simulink model "Line_keeping"  (R2023a)
settings: Solver=ode23tb  StartTime=0.0  StopTime=50  RelTol=1e-3
model workspace (MAT data in the model file):
  BusActorsActors = canlib.Parameter
  BusActorsActors.DataType = 'auto'
  BusActorsActors.Complexity = 'real'
  BusActorsActors.Dimensions = [0 0]
values from neighbouring files (symbols this model uses):
  Cf = 19000    [L_1_init.m]    (also in calc_KMax.m; calc_Kmin.m; init.m; init_h2.m)
  Cr = 33000    [L_1_init.m]    (also in calc_KMax.m; calc_Kmin.m; init.m; init_h2.m)
  Iz = 2875    [L_1_init.m]    (also in calc_KMax.m; calc_Kmin.m; init.m; init_h2.m)
  Lf = 1.2    [L_1_init.m]    (also in calc_KMax.m; calc_Kmin.m; init.m; init_h2.m)
  Lr = 1.6    [L_1_init.m]    (also in calc_KMax.m; calc_Kmin.m; init.m; init_h2.m)
  m = dim(2)    [H_2_gain.m]    (also in L_1_init.m = 1575; calc_KMax.m = 1575; calc_Kmin.m = 1575; init.m = 1575)
  x_0 = [0 0 0 0]'    [L_1_init.m]    (also in init.m; init_h2.m; init_h8.m)
undefined symbols (not defined in the file or in its folder): driving, sigbuilder_block
libraries: drivingscenarioandsensors x2
settings Model: PacingRate=2  Creator=Utente  LastModifiedBy=csanc
settings SolverCC: AlgebraicLoopSolver=TrustRegion
settings DebuggingCC: UnconnectedInputMsg=warning  UnconnectedOutputMsg=warning  UnconnectedLineMsg=warning
settings ModelReferenceCC: EnableRefExpFcnMdlSchedulingChecks=on
settings RTWCC: DLArmComputeVersion=19.05

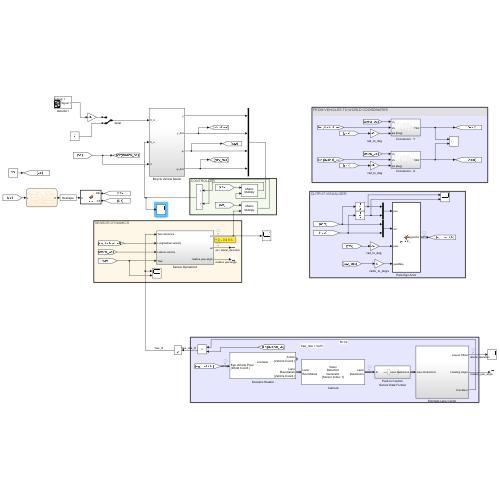
[thumbnail: Simulink's stored preview of the top-level diagram]
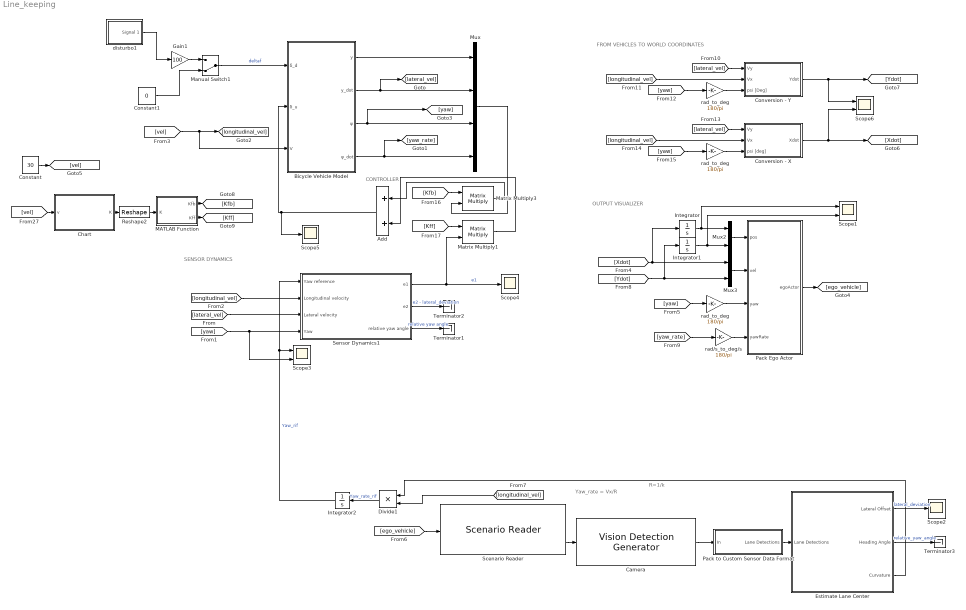
== system Line_keeping ==
  note: R=1/k
  note: Yaw_rate = Vx/R
  note: FROM VEHICLES TO WORLD COORDINATES
  note: SENSOR DYNAMICS
  note: CONTROLLER
  note: OUTPUT VISUALIZER
  Add : Sum
  Bicycle Vehicle Model : Subsystem
  Camera : drivingscenarioandsensors/Vision Detection Generator  SensorIndex=1  DetectorOutput=Lanes only  UpdateInterval=0.1  LaneUpdateInterval=0.01  SensorLocation=[1.9 0]  Height=1.1  Yaw=0  Pitch=0  Roll=0  BusNameSource=Auto  BusName=BusObjectDetections  BusName2Source=Property  BusName2=BusVision  MaxNumDetectionsSource=Property  MaxNumDetections=50  MaxNumLanesSource=Property  MaxNumLanes=2  DetectionCoordinates=Ego Cartesian  SimulateUsing=Interpreted execution  MaxRange=50  BoundingBoxAccuracy=10  ProcessNoiseIntensity=5  MaxSpeed=50  MaxAllowedOcclusion=0.5  MinObjectImageSize=[15 15]  DetectionProbability=0.9  FalsePositivesPerImage=0.1  MinLaneImageSize=[20 3]  LaneBoundaryAccuracy=3  HasNoise=on  InitialSeedSource=Repeatable  InitialSeed=0  UsedSeed=0  ActorProfilesSource=Parameters  ActorProfilesParameters=driving.internal.ActorProfilesParameters  ActorProfilesExpression=[struct('ActorID',1,'ClassID',1,'Length',4.7,'Width',1.8,'Height',1.4,'OriginOffset',[-1.35 0 0],'MeshVertices',[3.7 -0.9 1.4;3.7 0.9 1.4;-1 0.9 1.4;-1 -0.9 1.4;3.7 -0.9 0;3.7 0.9 0;-1 0.9 0;-1 -0.9 0],'MeshFaces',[6 2 1;1 5 6;8 4 3;3 7 8;6 7 3;3 2 6;5 1 4;4 8 5;4 1 2;2 3 4;7 6 5;5 8 7],'RCSPattern',[10 10;10 10],'RCSAzimuthAngles',[-180 180],'RCSElevationAngles',[-90 90])]  Intrinsics=driving.internal.cameraIntrinsics('FocalLength',[800 800],'PrincipalPoint',[320 240],'ImageSize',[480 640],'RadialDistortion',[0 0],'TangentialDistortion',[0 0],'Skew',0)
  Chart : Stateflow chart  TreatAsAtomicUnit=on
  Constant : Constant  Value=30
  Constant1 : Constant  Value=0
  Conversion - X : Subsystem
  Conversion - Y : Subsystem
  Divide1 : Product  Inputs=**
  Estimate Lane Center : Subsystem  VariantControl=v2
  Gain1 : Gain  Gain=100
  Integrator : Integrator
  Integrator1 : Integrator  InitialCondition=-0.02
  Integrator2 : Integrator
  MATLAB Function : MATLAB Function  TreatAsAtomicUnit=on
  Manual Switch1 : ManualSwitch  CurrentSetting=0
  Matrix Multiply1 : Product  Multiplication=Matrix(*)
  Matrix Multiply3 : Product  Multiplication=Matrix(*)
  Mux : Mux
  Mux2 : Mux  Inputs=2
  Mux3 : Mux  Inputs=2
  Pack Ego Actor : MATLAB Function  TreatAsAtomicUnit=on
  Pack to Custom Sensor Data Format : Subsystem
  Reshape2 : Reshape  OutputDimensionality=Customize  OutputDimensions=[1,5]
  Scenario Reader : drivingscenarioandsensors/Scenario Reader  ScenarioSource=From file  ScenarioFileName=D:\Proyecto_vehicle_control\modulo 2\scenario.mat  ScenarioVariableName=scenario  OutputCoordinateSystem=Vehicle coordinates  EgoVehicleSource=Input port  EgoVehicleActorID=1  OrientVehiclesOnRoad=off  OutputEgoVehiclePose=off  OutputEgoVehicleState=off  SampleTime=.1  LaneBoundaryOutput=Ego vehicle lane boundaries  LaneBoundaryDistance=linspace(-150, 150, 101)  LaneBoundaryLocation=Center of lane markings  BusNameSource=Auto  BusName=BusActors  BusNumActorsSource=Scenario  BusNumActors=100  BusName2Source=Auto  BusName2=BusLaneBoundaries  BusNumLaneBoundariesSource=Scenario  BusNumLaneBoundaries=10  BusName3Source=Auto  BusName3=BusEgoActor  BusName4Source=Auto  BusName4=BusEgoState  ShowCoordinateLabels=on  SimulateUsing=Interpreted execution
  Scope1 : Scope  NumInputPorts=2
  Scope2 : Scope
  Scope3 : Scope  NumInputPorts=2
  Scope4 : Scope
  Scope5 : Scope
  Scope6 : Scope  NumInputPorts=2
  Sensor Dynamics1 : Subsystem
  Terminator1 : Terminator
  Terminator2 : Terminator
  Terminator3 : Terminator
  disturbo1 : Subsystem  Tag=STV Subsys  LoadFcn=sigbuilder_block('load');  StartFcn=sigbuilder_block('start');  StopFcn=sigbuilder_block('stop');  ClipboardFcn=sigbuilder_block('clipboard');  mask(Sigbuilder block){tuvar=[0:10]}
      mask help: Simulink:masks:SigbuilderBlock_MD
      mask init:
      | if ~strcmp(get_param(bdroot(gcbh),'SimulationStatus'),'stopped') tuvar = sigbuilder_block('maskInit'); end
      settings: CopyFcn=sigbuilder_block('copy');  DeleteFcn=sigbuilder_block('delete');  ModelCloseFcn=sigbuilder_block('modelClose');  PreSaveFcn=sigbuilder_block('preSave');  PauseFcn=sigbuilder_block('pause');  ContinueFcn=sigbuilder_block('continue');  NameChangeFcn=sigbuilder_block('namechange');  OpenFcn=sigbuilder_block('open',[406.2 255 401.4 229.8 ]);  CloseFcn=sigbuilder_block('close');
      mask Display: plot(0, 0, 100, 100,[2, 2, 32, 32, 2], [68, 8, 8, 68, 68],[32, 2], [38, 38], [32, 19, 2],[53, 60, 44], [32, 17, 17, 2],[16, 16, 31, 31]);txt = getActiveGroup(gcbh);text(2, 100, txt,'verticalAlignment', 'top');
  rad/s_to_deg/s : Gain  Gain=180/pi
  rad_to_deg : Gain  Gain=180/pi
  "rad_to_deg " : Gain  Gain=180/pi
  "rad_to_deg  " : Gain  Gain=180/pi
  wires:
  Bicycle Vehicle Model/1(y) -> Mux/1
  Bicycle Vehicle Model/2(y_dot) -> [lateral_vel], Mux/2
  Bicycle Vehicle Model/4(ψ_dot) -> [yaw_rate], Mux/4
  Mux/1 -> Matrix Multiply3/2
  [longitudinal_vel] -> Sensor Dynamics1/2(Longitudinal velocity)
  [lateral_vel] -> Sensor Dynamics1/3(Lateral velocity)
  [yaw] -> Scope3/2, Sensor Dynamics1/4("Yaw ")
  Mux2/1 -> Pack Ego Actor/1(pos)
  [Xdot] -> Integrator/1, Mux3/1
  Mux3/1 -> Pack Ego Actor/2(vel)
  [yaw] -> "rad_to_deg  "/1
  Pack Ego Actor/1(egoActor) -> [ego_vehicle]
  [yaw_rate] -> rad/s_to_deg/s/1
  "rad_to_deg  "/1 -> Pack Ego Actor/3(yaw)
  [Ydot] -> Integrator1/1, Mux3/2
  rad/s_to_deg/s/1 -> Pack Ego Actor/4(yawRate)
  [lateral_vel] -> Conversion - Y/1(Vy)
  [longitudinal_vel] -> Conversion - Y/2(Vx)
  Conversion - X/1(Xdot) -> [Xdot], Scope6/2
  [yaw] -> rad_to_deg/1
  [yaw] -> "rad_to_deg "/1
  [longitudinal_vel] -> Conversion - X/2(Vx)
  [lateral_vel] -> Conversion - X/1(Vy)
  rad_to_deg/1 -> Conversion - X/3(psi [deg])
  "rad_to_deg "/1 -> Conversion - Y/3(psi [Deg])
  Sensor Dynamics1/3(relative yaw angle) -> Terminator1/1  "relative yaw angle"
  Integrator/1 -> Scope1/1, Mux2/1
  Integrator1/1 -> Scope1/2, Mux2/2
  Camera/1 -> Pack to Custom Sensor Data Format/1(In)
  Scenario Reader/2 -> Camera/1
  Pack to Custom Sensor Data Format/1(Lane Detections) -> Estimate Lane Center/1(Lane Detections)
  [ego_vehicle] -> Scenario Reader/1
  Divide1/1 -> Integrator2/1  "Yaw_rate_rif"
  Add/1 -> Scope5/1, Bicycle Vehicle Model/2(δ_u)
  Bicycle Vehicle Model/3(ψ) -> [yaw], Mux/3
  Estimate Lane Center/3(" Curvature") -> Divide1/1
  Conversion - Y/1(Ydot) -> [Ydot], Scope6/1
  Integrator2/1 -> Scope3/1, Sensor Dynamics1/1(Yaw reference)  "Yaw_rif"
  [longitudinal_vel] -> Divide1/2
  Sensor Dynamics1/2(e2) -> Terminator2/1  "e2 - lateral_deviation"
  Estimate Lane Center/1(Lateral Offset) -> Scope2/1  "lateral_deviation"
  [vel] -> Chart/1(v)
  [vel] -> [longitudinal_vel], Bicycle Vehicle Model/3(V)
  MATLAB Function/1(Kfb) -> [Kfb]
  MATLAB Function/2(Kff) -> [Kff]
  [Kfb] -> Matrix Multiply3/1
  Matrix Multiply3/1 -> Add/1
  [Kff] -> Matrix Multiply1/1
  Sensor Dynamics1/1(e1) -> Scope4/1, Matrix Multiply1/2  "e1"
  Matrix Multiply1/1 -> Add/2
  Chart/1(K) -> Reshape2/1
  Reshape2/1 -> MATLAB Function/1(K)
  Constant/1 -> [vel]
  Constant1/1 -> Manual Switch1/2
  Manual Switch1/1 -> Bicycle Vehicle Model/1(δ_d)  "deltaf"
  disturbo1/1(Signal 1) -> Gain1/1
  Gain1/1 -> Manual Switch1/1
  Estimate Lane Center/2(Heading Angle) -> Terminator3/1  "relative_yaw_angle"

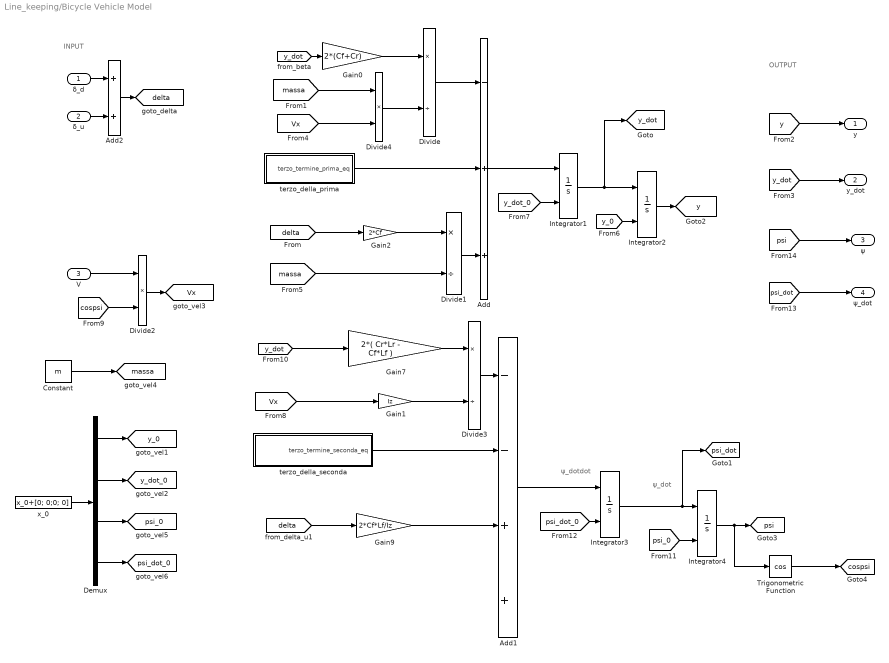
== system Line_keeping/Bicycle Vehicle Model ==
  note: ψ_dot
  note: OUTPUT
  note: INPUT
  note: ψ_dotdot
  δ_d : Inport
  δ_u : Inport  Port=2
  V : Inport  Port=3
  Add : Sum  Inputs=-++
  Add1 : Sum  Inputs=--++
  Add2 : Sum
  Constant : Constant  Value=m
  Demux : Demux
  Divide : Product  Inputs=*/
  Divide1 : Product  Inputs=*/
  Divide2 : Product  Inputs=**
  Divide3 : Product  Inputs=*/
  Divide4 : Product  Inputs=**
  Gain0 : Gain  Gain=2*(Cf+Cr)
  Gain1 : Gain  Gain=Iz
  Gain2 : Gain  Gain=2*Cf
  Gain7 : Gain  Gain="2*( Cr*Lr  - Cf*Lf )"
  Gain9 : Gain  Gain=2*Cf*Lf/Iz
  Integrator1 : Integrator  InitialConditionSource=external
  Integrator2 : Integrator  InitialConditionSource=external
  Integrator3 : Integrator  InitialConditionSource=external
  Integrator4 : Integrator  InitialConditionSource=external  LowerSaturationLimit=0
  Trigonometric Function : Trigonometry  Operator=cos
  terzo_della_prima : Subsystem
  terzo_della_seconda : Subsystem
  "x_0 " : Constant  Value=x_0+[0; 0;0; 0]
  y : Outport
  y_dot : Outport  Port=2
  ψ : Outport  Port=3
  ψ_dot : Outport  Port=4
  tag scope: Vx=global, cospsi=global, delta=global, massa=global, psi=global, psi_0=global, psi_dot=global, psi_dot_0=global, y=global, y_0=global, y_dot=global, y_dot_0=global
  wires:
  [psi] -> ψ/1
  [psi_dot] -> ψ_dot/1
  [psi_dot_0] -> Integrator3/2
  [psi_0] -> Integrator4/2
  [cospsi] -> Divide2/2
  Trigonometric Function/1 -> [cospsi]
  Divide2/1 -> [Vx]
  Integrator4/1 -> [psi], Trigonometric Function/1
  [Vx] -> Gain1/1
  Gain1/1 -> Divide3/2
  Divide3/1 -> Add1/1
  [y_0] -> Integrator2/2
  [y_dot_0] -> Integrator1/2
  Demux/4 -> [psi_dot_0]
  Demux/3 -> [psi_0]
  Integrator2/1 -> [y]
  Integrator1/1 -> [y_dot], Integrator2/1
  Divide1/1 -> Add/3
  [massa] -> Divide1/2
  Divide/1 -> Add/1
  [Vx] -> Divide4/2
  [massa] -> Divide4/1
  Divide4/1 -> Divide/2
  "x_0 "/1 -> Demux/1
  [delta] -> Gain2/1
  Add2/1 -> [delta]
  Gain9/1 -> Add1/3
  terzo_della_seconda/1("terzo_termine_seconda_eq ") -> Add1/2
  Gain2/1 -> Divide1/1
  terzo_della_prima/1("terzo_termine_prima_eq ") -> Add/2
  Demux/2 -> [y_dot_0]
  Demux/1 -> [y_0]
  Constant/1 -> [massa]
  Integrator3/1 -> Integrator4/1, [psi_dot]
  Add/1 -> Integrator1/1
  [y_dot] -> Gain7/1
  [y_dot] -> Gain0/1
  [y_dot] -> y_dot/1
  [y] -> y/1
  [delta] -> Gain9/1
  Gain7/1 -> Divide3/1
  Add1/1 -> Integrator3/1
  Gain0/1 -> Divide/1
  V/1 -> Divide2/1
  δ_u/1 -> Add2/2
  δ_d/1 -> Add2/1

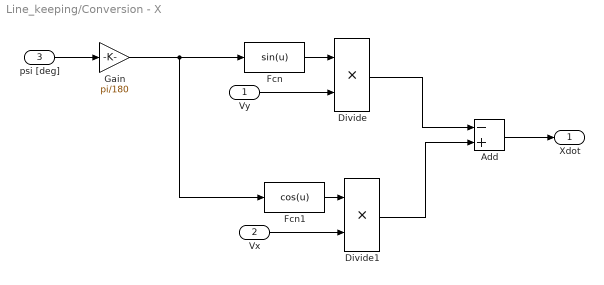
== system Line_keeping/Conversion - X ==
  Vy : Inport
  Vx : Inport  Port=2
  psi [deg] : Inport  Port=3
  Add : Sum  Inputs=-+
  Divide : Product  Inputs=**
  Divide1 : Product  Inputs=**
  Fcn : Fcn  Expr=sin(u)
  Fcn1 : Fcn  Expr=cos(u)
  Gain : Gain  Gain=pi/180
  Xdot : Outport
  wires:
  Gain/1 -> Fcn/1, Fcn1/1
  Add/1 -> Xdot/1
  Divide1/1 -> Add/2
  Vx/1 -> Divide1/2
  Fcn1/1 -> Divide1/1
  Divide/1 -> Add/1
  Vy/1 -> Divide/2
  Fcn/1 -> Divide/1
  psi [deg]/1 -> Gain/1

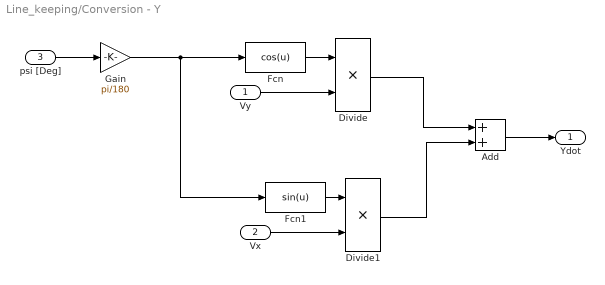
== system Line_keeping/Conversion - Y ==
  Vy : Inport
  Vx : Inport  Port=2
  psi [Deg] : Inport  Port=3
  Add : Sum
  Divide : Product  Inputs=**
  Divide1 : Product  Inputs=**
  Fcn : Fcn  Expr=cos(u)
  Fcn1 : Fcn  Expr=sin(u)
  Gain : Gain  Gain=pi/180
  Ydot : Outport
  wires:
  psi [Deg]/1 -> Gain/1
  Fcn/1 -> Divide/1
  Vy/1 -> Divide/2
  Divide/1 -> Add/1
  Fcn1/1 -> Divide1/1
  Vx/1 -> Divide1/2
  Divide1/1 -> Add/2
  Add/1 -> Ydot/1
  Gain/1 -> Fcn1/1, Fcn/1

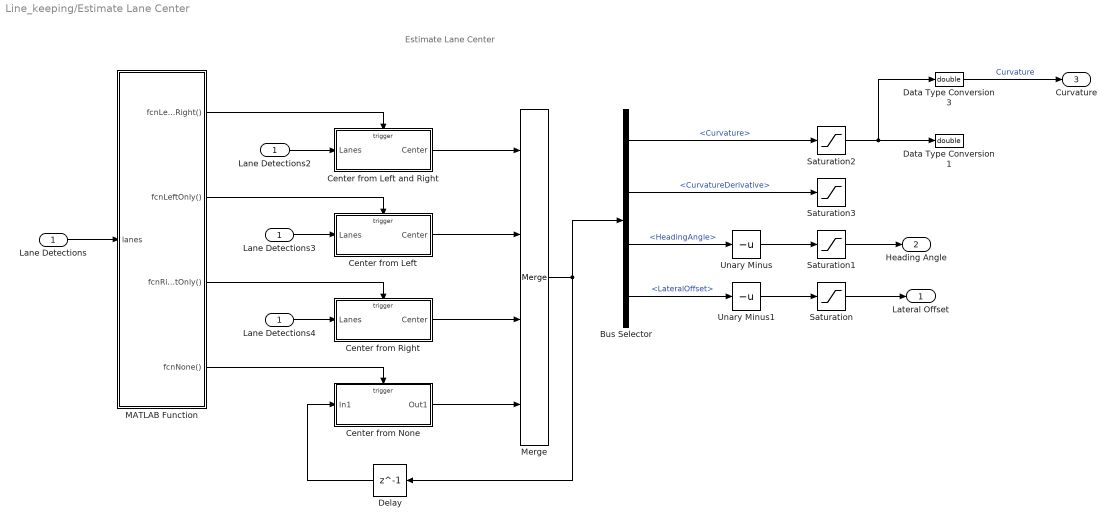
== system Line_keeping/Estimate Lane Center ==
  note: Estimate Lane Center
  Lane Detections : Inport
  Bus Selector : BusSelector  OutputSignals=Curvature,CurvatureDerivative,HeadingAngle,LateralOffset
  Center from Left : Subsystem  TreatAsAtomicUnit=on
  Center from Left and Right : Subsystem  TreatAsAtomicUnit=on
  Center from None : Subsystem  TreatAsAtomicUnit=on
  Center from Right : Subsystem  TreatAsAtomicUnit=on
  Data Type Conversion1 : DataTypeConversion  OutDataTypeStr=double  SaturateOnIntegerOverflow=off  RndMeth=Floor
  Data Type Conversion3 : DataTypeConversion  OutDataTypeStr=double  SaturateOnIntegerOverflow=off  RndMeth=Floor
  Delay : Delay  DelayLength=1
  Lane Detections2 : InportShadow
  Lane Detections3 : InportShadow
  Lane Detections4 : InportShadow
  MATLAB Function : MATLAB Function  TreatAsAtomicUnit=on
  Merge : Merge  Inputs=4
  Saturation : Saturate  UpperLimit=inf
  Saturation1 : Saturate  UpperLimit=0.6  LowerLimit=-0.6
  Saturation2 : Saturate  UpperLimit=0.15  LowerLimit=-0.15
  Saturation3 : Saturate  UpperLimit=0.15  LowerLimit=-0.15
  Unary Minus : UnaryMinus
  Unary Minus1 : UnaryMinus
  Lateral Offset : Outport  VectorParamsAs1DForOutWhenUnconnected=off
  Heading Angle : Outport  Port=2  VectorParamsAs1DForOutWhenUnconnected=off
  " Curvature" : Outport  Port=3  VectorParamsAs1DForOutWhenUnconnected=off
  wires:
  Center from Right/1(Center) -> Merge/3
  Lane Detections3/1 -> Center from Left/1(Lanes)
  Lane Detections4/1 -> Center from Right/1(Lanes)
  MATLAB Function/2(fcnLeftOnly()) -> Center from Left/Trigger
  Center from None/1(Out1) -> Merge/4
  MATLAB Function/1(fcnLeftAndRight()) -> Center from Left and Right/Trigger
  Delay/1 -> Center from None/1(In1)
  Center from Left and Right/1(Center) -> Merge/1
  Lane Detections/1 -> MATLAB Function/1(lanes)
  Lane Detections2/1 -> Center from Left and Right/1(Lanes)
  MATLAB Function/3(fcnRightOnly()) -> Center from Right/Trigger
  MATLAB Function/4(fcnNone()) -> Center from None/Trigger
  Center from Left/1(Center) -> Merge/2
  Merge/1 -> Bus Selector/1, Delay/1
  Saturation2/1 -> Data Type Conversion1/1, Data Type Conversion3/1
  Saturation1/1 -> Heading Angle/1
  Saturation/1 -> Lateral Offset/1
  Unary Minus/1 -> Saturation1/1
  Bus Selector/2 -> Saturation3/1  "<CurvatureDerivative>"
  Bus Selector/1 -> Saturation2/1  "<Curvature>"
  Unary Minus1/1 -> Saturation/1
  Bus Selector/4 -> Unary Minus1/1  "<LateralOffset>"
  Bus Selector/3 -> Unary Minus/1  "<HeadingAngle>"
  Data Type Conversion3/1 -> " Curvature"/1  "Curvature"

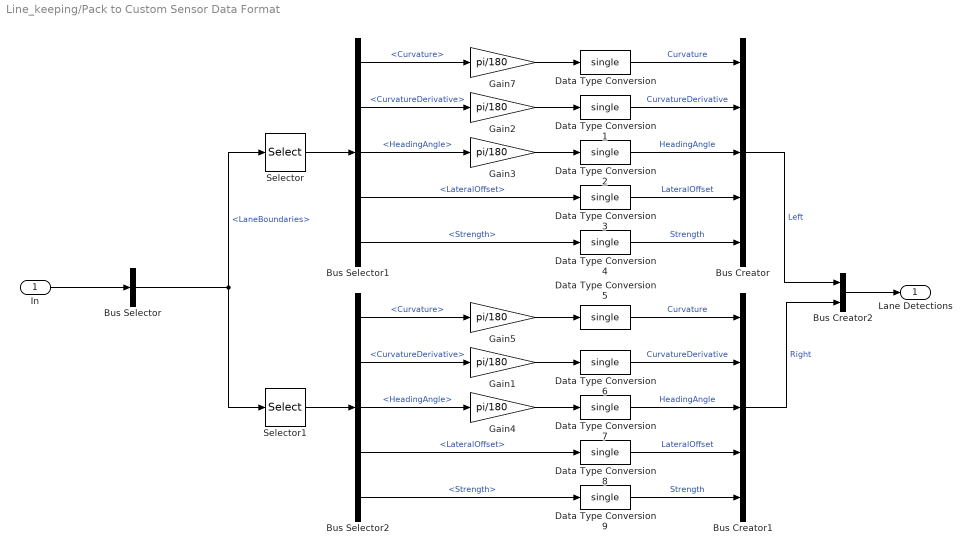
== system Line_keeping/Pack to Custom Sensor Data Format ==
  In : Inport
  Bus Creator : BusCreator  Inputs=5  OutDataTypeStr=Bus: LaneSensorBoundaries
  Bus Creator1 : BusCreator  Inputs=5  OutDataTypeStr=Bus: LaneSensorBoundaries
  Bus Creator2 : BusCreator  Inputs=2  OutDataTypeStr=Bus: LaneSensor
  Bus Selector : BusSelector  OutputSignals=LaneBoundaries
  Bus Selector1 : BusSelector  OutputSignals=Curvature,CurvatureDerivative,HeadingAngle,LateralOffset,Strength
  Bus Selector2 : BusSelector  OutputSignals=Curvature,CurvatureDerivative,HeadingAngle,LateralOffset,Strength
  Data Type Conversion{,1..9} (10 alike) : DataTypeConversion  OutDataTypeStr=single  SaturateOnIntegerOverflow=off  RndMeth=Floor
  Gain{1..5,7} (6 alike) : Gain  Gain=pi/180
  Selector : Selector  InputPortWidth=2  IndexOptions=Index vector (dialog)  Indices=1  OutputSizes=1
  Selector1 : Selector  InputPortWidth=2  IndexOptions=Index vector (dialog)  Indices=2  OutputSizes=1
  Lane Detections : Outport  VectorParamsAs1DForOutWhenUnconnected=off
  wires:
  In/1 -> Bus Selector/1
  Bus Selector/1 -> Selector/1, Selector1/1  "<LaneBoundaries>"
  Selector/1 -> Bus Selector1/1
  Bus Selector1/2 -> Gain2/1  "<CurvatureDerivative>"
  Bus Selector1/1 -> Gain7/1  "<Curvature>"
  Bus Selector1/3 -> Gain3/1  "<HeadingAngle>"
  Gain7/1 -> Data Type Conversion/1
  Gain2/1 -> Data Type Conversion1/1
  Gain3/1 -> Data Type Conversion2/1
  Bus Selector1/4 -> Data Type Conversion3/1  "<LateralOffset>"
  Bus Selector1/5 -> Data Type Conversion4/1  "<Strength>"
  Data Type Conversion/1 -> Bus Creator/1  "Curvature"
  Data Type Conversion1/1 -> Bus Creator/2  "CurvatureDerivative"
  Data Type Conversion2/1 -> Bus Creator/3  "HeadingAngle"
  Data Type Conversion3/1 -> Bus Creator/4  "LateralOffset"
  Data Type Conversion4/1 -> Bus Creator/5  "Strength"
  Data Type Conversion9/1 -> Bus Creator1/5  "Strength"
  Data Type Conversion6/1 -> Bus Creator1/2  "CurvatureDerivative"
  Data Type Conversion7/1 -> Bus Creator1/3  "HeadingAngle"
  Data Type Conversion8/1 -> Bus Creator1/4  "LateralOffset"
  Data Type Conversion5/1 -> Bus Creator1/1  "Curvature"
  Bus Selector2/1 -> Gain5/1  "<Curvature>"
  Selector1/1 -> Bus Selector2/1
  Bus Selector2/4 -> Data Type Conversion8/1  "<LateralOffset>"
  Bus Selector2/5 -> Data Type Conversion9/1  "<Strength>"
  Bus Selector2/2 -> Gain1/1  "<CurvatureDerivative>"
  Gain4/1 -> Data Type Conversion7/1
  Gain5/1 -> Data Type Conversion5/1
  Gain1/1 -> Data Type Conversion6/1
  Bus Selector2/3 -> Gain4/1  "<HeadingAngle>"
  Bus Creator2/1 -> Lane Detections/1
  Bus Creator/1 -> Bus Creator2/1  "Left"
  Bus Creator1/1 -> Bus Creator2/2  "Right"

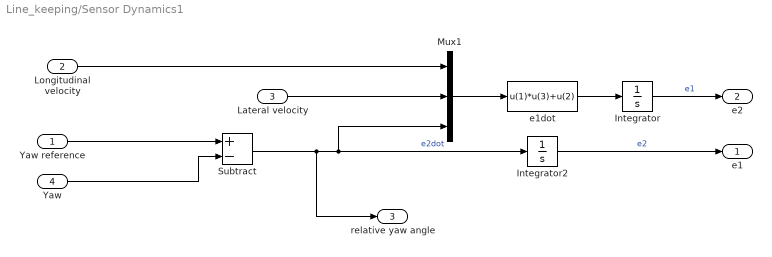
== system Line_keeping/Sensor Dynamics1 ==
  Yaw reference : Inport
  Longitudinal velocity : Inport  Port=2
  Lateral velocity : Inport  Port=3
  "Yaw " : Inport  Port=4
  Integrator : Integrator
  Integrator2 : Integrator
  Mux1 : Mux  Inputs=[1 1 1]
  Subtract : Sum  Inputs=+-
  e1dot : Fcn  Expr=u(1)*u(3)+u(2)
  e1 : Outport  VectorParamsAs1DForOutWhenUnconnected=off
  e2 : Outport  Port=2  VectorParamsAs1DForOutWhenUnconnected=off
  relative yaw angle : Outport  Port=3  VectorParamsAs1DForOutWhenUnconnected=off
  wires:
  Integrator2/1 -> e1/1  "e2"
  Mux1/1 -> e1dot/1
  e1dot/1 -> Integrator/1
  Longitudinal velocity/1 -> Mux1/1
  Lateral velocity/1 -> Mux1/2
  Integrator/1 -> e2/1  "e1"
  Yaw reference/1 -> Subtract/1
  "Yaw "/1 -> Subtract/2
  Subtract/1 -> relative yaw angle/1, Mux1/3, Integrator2/1  "e2dot"

== system Line_keeping/disturbo1 ==
  Demux : Demux  Tag=STV Demux  Outputs=1
      settings: DisplayOption=none
  FromWs : FromWorkspace  Tag=STV FromWs  VariableName=tuvar
      SigBuilderData=|
      | common.afterFinalStr = 'Extrapolate'
      | common.sampleTime = 0
      | dataSet.timeRange = [0 22]
      | dataSet.name = 'Group 1'
      | sbobj.Groups.Name = 'Group 1'
      | sbobj.Groups.Signals.Name = 'Signal 1'
      | sbobj.Groups.Signals.XData = [0 0.105263157895 0.210526315789 0.315789473684 0.421052631579 0.526315789474 0.631578947368 0.736842105263 0.842105263158 0.947368421053 1.05263157895 1.15789473684 1.26315789474 1.36842105263 1.47368421053 1.57894736842 1.68421052632 1.78947368421 1.89473684211 2 2.10526315789 2.21052631579 2.31578947368 2.42105263158 2.52631578947 2.63157894737 2.73684210526 2.84210526316 2.94736842105 3.05263157895 3.15789473684 3.26315789474 3.36842105263 3.47368421053 3.57894736842 3.68421052632 3.78947368421 3.89473684211 4 4.10526315789 4.21052631579 4.31578947368 4.42105263158 4.52631578947 4.63157894737 4.73684210526 4.84210526316 4.94736842105 5.05263157895 5.15789473684 5.26315789474 5.36842105263 5.47368421053 5.57894736842 5.68421052632 5.78947368421 5.89473684211 6 6.10526315789 6.21052631579 6.31578947368 6.42105263158 6.52631578947 6.63157894737 6.73684210526 6.84210526316 6.94736842105 7.05263157895 7.15789473684 7.26315789474 7.36842105263 7.47368421053 7.57894736842 22]
      | sbobj.Groups.Signals.YData = [0 0 0 0 0.6 0.92 0.7 0 -0.82 -0.88 -0.78 0 0.42 0.48 0 0 0 0 0 0 0 0 0 0 0 0 0 0 0 0 0 0 0 0 0 0 0 0 0 0.02 0 0 0 -0.02 0 0.56 0.74 0.66 0 -0.59 -0.67 -0.53 0.78 0.72 0 0 0 0 0 0 0 0 0 0 0 0 0 0 0 0 0 0 0 0]
      | sbobj.Groups.TimeRange = [0 22]
  Signal 1 : Outport  Tag=STV Outport
  wires:
  Demux/1 -> Signal 1/1
  FromWs/1 -> Demux/1

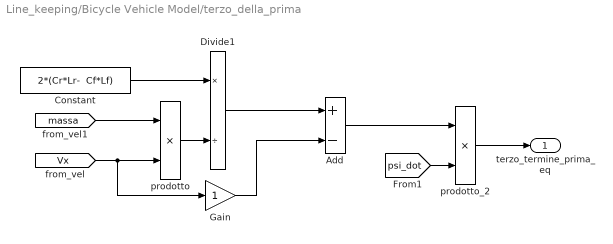
== system Line_keeping/Bicycle Vehicle Model/terzo_della_prima ==
  Add : Sum  Inputs=+-
  Constant : Constant  Value="2*(Cr*Lr-  Cf*Lf)"
  Divide1 : Product  Inputs=*/
  Gain : Gain
  prodotto : Product  Inputs=**
  prodotto_2 : Product  Inputs=**
  "terzo_termine_prima_eq " : Outport
  wires:
  Gain/1 -> Add/2
  [massa] -> prodotto/1
  prodotto/1 -> Divide1/2
  Add/1 -> prodotto_2/1
  [Vx] -> prodotto/2, Gain/1
  prodotto_2/1 -> "terzo_termine_prima_eq "/1
  [psi_dot] -> prodotto_2/2
  Divide1/1 -> Add/1
  Constant/1 -> Divide1/1

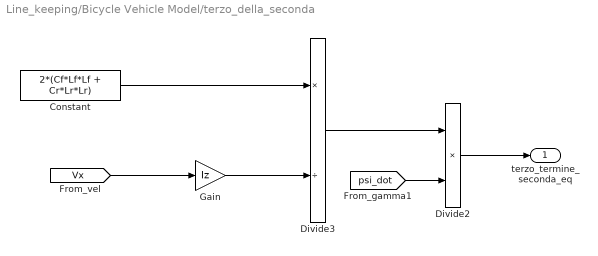
== system Line_keeping/Bicycle Vehicle Model/terzo_della_seconda ==
  Constant : Constant  Value=2*(Cf*Lf*Lf + Cr*Lr*Lr)
  Divide2 : Product  Inputs=**
  Divide3 : Product  Inputs=*/
  Gain : Gain  Gain=Iz
  "terzo_termine_seconda_eq " : Outport
  wires:
  Divide2/1 -> "terzo_termine_seconda_eq "/1
  [psi_dot] -> Divide2/2
  Gain/1 -> Divide3/2
  [Vx] -> Gain/1
  Divide3/1 -> Divide2/1
  Constant/1 -> Divide3/1

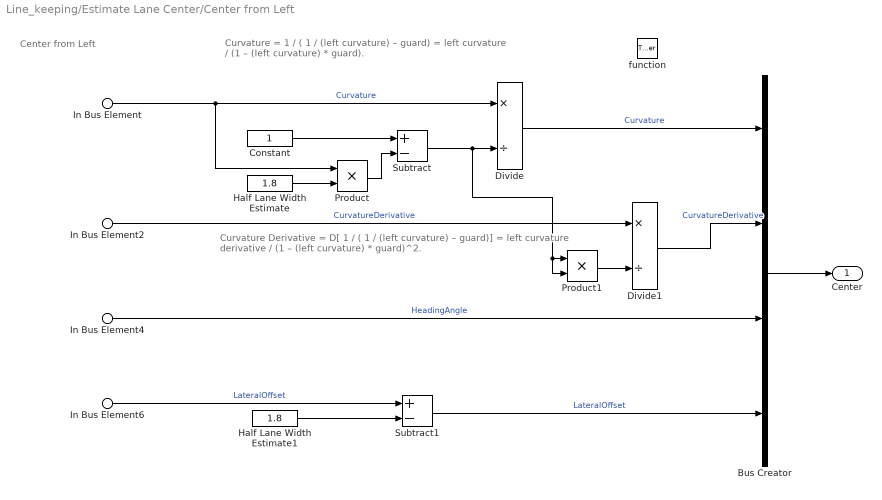
== system Line_keeping/Estimate Lane Center/Center from Left ==
  note: Curvature Derivative
      | = D[ 1 / ( 1 / (left curvature) – guard)]
      | = left curvature derivative / (1 – (left curvature) * guard)^2.
  note: Center from Left
  note: Curvature
      | = 1 / ( 1 / (left curvature) – guard)
      | = left curvature / (1 – (left curvature) * guard).
  In Bus Element : Inport  PortName=Lanes  Element=Left.Curvature
  In Bus Element2 : Inport  PortName=Lanes  Element=Left.CurvatureDerivative
  In Bus Element4 : Inport  PortName=Lanes  Element=Left.HeadingAngle
  In Bus Element6 : Inport  PortName=Lanes  Element=Left.LateralOffset
  function : TriggerPort  TriggerType=function-call  VariantControl=Variant
  Bus Creator : BusCreator  Inputs=4
  Constant : Constant  OutDataTypeStr=Inherit: Inherit via back propagation
  Divide : Product  Inputs=*/
  Divide1 : Product  Inputs=*/
  Half Lane Width Estimate : Constant  Value=1.8  OutDataTypeStr=Inherit: Inherit via back propagation
  Half Lane Width Estimate1 : Constant  Value=1.8  OutDataTypeStr=Inherit: Inherit via back propagation
  Product : Product
  Product1 : Product
  Subtract : Sum  Inputs=+-
  Subtract1 : Sum  Inputs=+-
  Center : Outport  VectorParamsAs1DForOutWhenUnconnected=off
  wires:
  Product/1 -> Subtract/2
  Half Lane Width Estimate1/1 -> Subtract1/2
  In Bus Element6/1 -> Subtract1/1  "LateralOffset"
  Product1/1 -> Divide1/2
  In Bus Element2/1 -> Divide1/1  "CurvatureDerivative"
  Constant/1 -> Subtract/1
  Half Lane Width Estimate/1 -> Product/2
  Subtract/1 -> Divide/2, Product1/1, Product1/2
  In Bus Element/1 -> Divide/1, Product/1  "Curvature"
  Subtract1/1 -> Bus Creator/4  "LateralOffset"
  In Bus Element4/1 -> Bus Creator/3  "HeadingAngle"
  Divide/1 -> Bus Creator/1  "Curvature"
  Divide1/1 -> Bus Creator/2  "CurvatureDerivative"
  Bus Creator/1 -> Center/1

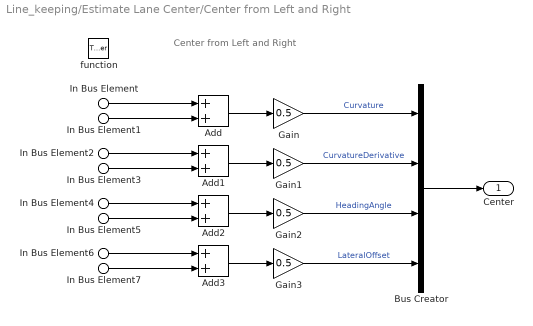
== system Line_keeping/Estimate Lane Center/Center from Left and Right ==
  note: Center from Left and Right
  In Bus Element : Inport  PortName=Lanes  Element=Left.Curvature
  In Bus Element2 : Inport  PortName=Lanes  Element=Left.CurvatureDerivative
  In Bus Element4 : Inport  PortName=Lanes  Element=Left.HeadingAngle
  In Bus Element6 : Inport  PortName=Lanes  Element=Left.LateralOffset
  In Bus Element1 : Inport  PortName=Lanes  Element=Right.Curvature
  In Bus Element3 : Inport  PortName=Lanes  Element=Right.CurvatureDerivative
  In Bus Element5 : Inport  PortName=Lanes  Element=Right.HeadingAngle
  In Bus Element7 : Inport  PortName=Lanes  Element=Right.LateralOffset
  function : TriggerPort  TriggerType=function-call  VariantControl=Variant
  Add{,1..3} (4 alike) : Sum
  Bus Creator : BusCreator  Inputs=4
  Gain{,1..3} (4 alike) : Gain  Gain=0.5
  Center : Outport  VectorParamsAs1DForOutWhenUnconnected=off
  wires:
  In Bus Element6/1 -> Add3/1
  In Bus Element7/1 -> Add3/2
  In Bus Element5/1 -> Add2/2
  In Bus Element4/1 -> Add2/1
  In Bus Element3/1 -> Add1/2
  In Bus Element2/1 -> Add1/1
  In Bus Element1/1 -> Add/2
  In Bus Element/1 -> Add/1
  Bus Creator/1 -> Center/1
  Gain3/1 -> Bus Creator/4  "LateralOffset"
  Add3/1 -> Gain3/1
  Gain2/1 -> Bus Creator/3  "HeadingAngle"
  Add2/1 -> Gain2/1
  Gain1/1 -> Bus Creator/2  "CurvatureDerivative"
  Add1/1 -> Gain1/1
  Gain/1 -> Bus Creator/1  "Curvature"
  Add/1 -> Gain/1

== system Line_keeping/Estimate Lane Center/Center from None ==
  In1 : Inport
  function : TriggerPort  TriggerType=function-call  VariantControl=Variant
  Out1 : Outport  VectorParamsAs1DForOutWhenUnconnected=off
  wires:
  In1/1 -> Out1/1

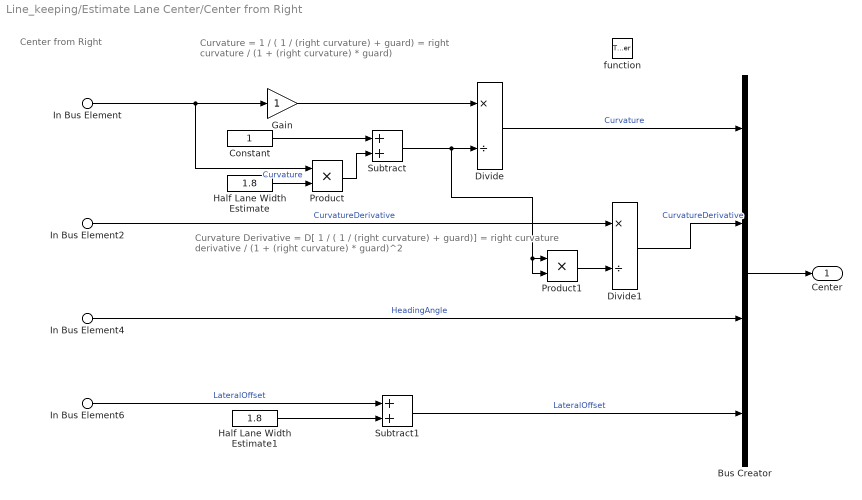
== system Line_keeping/Estimate Lane Center/Center from Right ==
  note: Curvature Derivative
      | = D[ 1 / ( 1 / (right curvature) + guard)]
      | = right curvature derivative / (1 + (right curvature) * guard)^2
  note: Curvature
      | = 1 / ( 1 / (right curvature) + guard)
      | = right curvature / (1 + (right curvature) * guard)
  note: Center from Right
  In Bus Element : Inport  PortName=Lanes  Element=Right.Curvature
  In Bus Element2 : Inport  PortName=Lanes  Element=Right.CurvatureDerivative
  In Bus Element4 : Inport  PortName=Lanes  Element=Right.HeadingAngle
  In Bus Element6 : Inport  PortName=Lanes  Element=Right.LateralOffset
  function : TriggerPort  TriggerType=function-call  VariantControl=Variant
  Bus Creator : BusCreator  Inputs=4
  Constant : Constant  OutDataTypeStr=Inherit: Inherit via back propagation
  Divide : Product  Inputs=*/
  Divide1 : Product  Inputs=*/
  Gain : Gain
  Half Lane Width Estimate : Constant  Value=1.8  OutDataTypeStr=Inherit: Inherit via back propagation
  Half Lane Width Estimate1 : Constant  Value=1.8  OutDataTypeStr=Inherit: Inherit via back propagation
  Product : Product
  Product1 : Product
  Subtract : Sum
  Subtract1 : Sum
  Center : Outport  VectorParamsAs1DForOutWhenUnconnected=off
  wires:
  Half Lane Width Estimate/1 -> Product/2
  Product/1 -> Subtract/2
  Constant/1 -> Subtract/1
  Subtract/1 -> Divide/2, Product1/1, Product1/2
  In Bus Element/1 -> Gain/1, Product/1  "Curvature"
  Bus Creator/1 -> Center/1
  Subtract1/1 -> Bus Creator/4  "LateralOffset"
  Divide/1 -> Bus Creator/1  "Curvature"
  In Bus Element6/1 -> Subtract1/1  "LateralOffset"
  Half Lane Width Estimate1/1 -> Subtract1/2
  In Bus Element4/1 -> Bus Creator/3  "HeadingAngle"
  Product1/1 -> Divide1/2
  Divide1/1 -> Bus Creator/2  "CurvatureDerivative"
  In Bus Element2/1 -> Divide1/1  "CurvatureDerivative"
  Gain/1 -> Divide/1

== matlab function Line_keeping/MATLAB Function ==
  data: K input; Kfb output; Kff output
function [Kfb,Kff]  = fcn(K)
Kfb = K(1,1:end-1);
Kff = K(1,5:end);
end

== matlab function Line_keeping/Pack Ego Actor ==
  data: pos input; egoActor output Bus: BusActors1Actors size=1; vel input; yaw input; yawRate input
function egoActor = packEgo(pos,vel,yaw,yawRate)
% Pack ego information into a single ego actor bus
%
% Imoprtant note:
% Output is a bus of type BusActorsActors. This is the same bus used by the
% Scenario Reader to output an individual actor. If you change the
% output bus name of Scenario Reader, change the output bus name here
% as well by clicking on 'Edit Data' in the menu above.

%Position x,y,z
%Velocity x,y,z
%Angular velocity wx, wy, wz

egoActor = struct(...
    'ActorID',1,...
    'Position', [pos(1) pos(2) 0], ...
    'Velocity', [vel(1) vel(2) 0], ...
    'Roll', 0, ...
    'Pitch', 0, ...
    'Yaw', yaw, ...
    'AngularVelocity', [0 0 yawRate]);

== matlab function Line_keeping/Estimate Lane Center/MATLAB Function ==
  data: lanes input
  events: fcnLeftAndRight output FUNCTION_CALL_EVENT; fcnLeftOnly output FUNCTION_CALL_EVENT; fcnRightOnly output FUNCTION_CALL_EVENT; fcnNone output FUNCTION_CALL_EVENT
function fcn(lanes)

leftStrength  = lanes.Left.Strength;
rightStrength = lanes.Right.Strength;

if (leftStrength > 0) && (rightStrength > 0)
   fcnLeftAndRight();
   
elseif leftStrength > 0
    fcnLeftOnly();
    
elseif rightStrength > 0
    fcnRightOnly();
    
else
    fcnNone();
end

== stateflow chart Line_keeping/Chart ==
  state S1
    entry: rho=(v-10)/(16-10);
    entry:Kmi=ml('calc_Kmin(%d%)',10);
    entry:KMa=ml('calc_KMax(%d%)',16);
    entry:K=(1-rho)*Kmi+rho*KMa;
    c1=v;
  state S4
    entry: rho=(v-28)/(34-28);
    entry:Kmi=ml('calc_Kmin(%d%)',28);
    entry:KMa=ml('calc_KMax(%d%)',34);
    entry:K=(1-rho)*Kmi+rho*KMa;
  note: Stato di neutro
  state S2
    entry: rho=(v-16)/(22-16);
    entry:Kmi=ml('calc_Kmin(%d%)',16);
    entry:KMa=ml('calc_KMax(%d%)',22);
    entry:K=(1-rho)*Kmi+rho*KMa;
    c1=v;
  state S0
  state S3
    entry: rho=(v-22)/(28-22);
    entry:Kmi=ml('calc_Kmin(%d%)',22);
    entry:KMa=ml('calc_KMax(%d%)',28);
    entry:K=(1-rho)*Kmi+rho*KMa;
  S0 -> S1 [order 1] : [v>10 && v<=16]
  S2 -> S1 [order 1] : [v<=16]
  S4 -> S3 : [v<=28]
  S1 -> S2 : [v>16]
  S0 -> S4 [order 2] : [v>28 && v<=34]
  S3 -> S4 [order 1] : [v>28]
  (default) -> S0
  S0 -> S2 [order 4] : [v>16 && v<=22]
  S0 -> S3 [order 3] : [v>22 && v<=28]
  S2 -> S3 [order 2] : [v>22]
  S3 -> S2 [order 2] : [v<=22]
  data: v input double; c1 local double; c2 local double; K output double size=5; Kmi local double size=5; KMa local double size=5; Kmi_2 local double size=4; KMa_2 local double size=4; Kmi_3 local double size=4; KMa_3 local double size=4; KMa_4 local double size=4; KMa_5 local double size=4; KMa_6 local double size=4; KMa_7 local double size=4; Kmi_4 local double size=4; Kmi_5 local double size=4; Kmi_6 local double size=4; Kmi_7 local double size=4; rho local double
